simulink model "Traffic_lights"  (R2020b)
settings: Solver=VariableStepAuto  StartTime=0.0  StopTime=200  RelTol=1e-3
settings Model: PacingRate=0.400000  Creator=Abhinav dixit  LastModifiedBy=Abhinav dixit

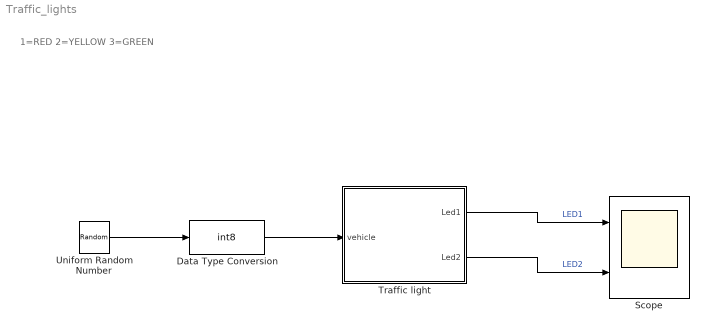
== system Traffic_lights ==
  note: 1=RED
      | 2=YELLOW
      | 3=GREEN
  Data Type Conversion : DataTypeConversion  OutDataTypeStr=int8  RndMeth=Nearest
  Scope : Scope  NumInputPorts=2
  Traffic light : Stateflow chart  TreatAsAtomicUnit=on
  Uniform Random Number : UniformRandomNumber  Minimum=0  Maximum=50  Seed=400  SampleTime=0
  wires:
  Data Type Conversion/1 -> Traffic light/1(vehicle)
  Uniform Random Number/1 -> Data Type Conversion/1
  Traffic light/1(Led1) -> Scope/1  "LED1"
  Traffic light/2(Led2) -> Scope/2  "LED2"

== stateflow chart Traffic_lights/Traffic light ==
  settings: stateMachineType=MOORE_MACHINE  initializeOutput=1
  state Stop
    Led1=RED;
    Led2=GREEN
  state StopForTraffic
    Led1=RED;
    Led2=GREEN;
  state Stoptogo
    Led1=RED;
    Led2=YELLOW;
  state GoToStop
    Led1=YELLOW;
    Led2=RED;
  state Go
    Led1=GREEN;
    Led2=RED;
  (default) -> Stop
  Stop -> StopForTraffic : after(20,tick)
  StopForTraffic -> Stoptogo : [vehicle>30]
  GoToStop -> Stop : after(3,tick)
  Stoptogo -> Go : after(3,tick)
  Go -> GoToStop : after(10,tick)
  data: Led1 output; Led2 output; RED constant double =1; GREEN constant double =3; YELLOW constant double =2; vehicle input
